simulink model "SPGF_FSK_0000_R2020b"  (R2020b)
settings: Solver=ode4  StartTime=0.0  StopTime=1.4  FixedStep=50e-6/50  RelTol=1e-3  EnableMultiTasking=on
undefined symbols (not defined in the file): D11, Delta
libraries: powerlib x2546, powerlib_meascontrol x183, simulink x24
(part 24 of 34)

== system SPGF_FSK_0000_R2020b/W35/concentrated ==
  Ccs/1 : powerlib/Elements/Series RLC Branch  LConnTagsString=__new0  RConnTagsString=__new0  BranchType=C  Resistance=190  Inductance=1e-3  SetiL0=off  InitialCurrent=0  Capacitance=-C_matrix(1,2)/2  Setx0=off  InitialVoltage=0  Measurements=None
  Ccs/2 : powerlib/Elements/Series RLC Branch  LConnTagsString=__new0  RConnTagsString=__new0  BranchType=C  Resistance=190  Inductance=1e-3  SetiL0=off  InitialCurrent=0  Capacitance=-C_matrix(1,2)/2  Setx0=off  InitialVoltage=0  Measurements=None
  Ccs2/1 : powerlib/Elements/Series RLC Branch  LConnTagsString=__new0  RConnTagsString=__new0  BranchType=C  Resistance=190  Inductance=1e-3  SetiL0=off  InitialCurrent=0  Capacitance=-C_matrix(3,4)/2  Setx0=off  InitialVoltage=0  Measurements=None
  Ccs2/2 : powerlib/Elements/Series RLC Branch  LConnTagsString=__new0  RConnTagsString=__new0  BranchType=C  Resistance=190  Inductance=1e-3  SetiL0=off  InitialCurrent=0  Capacitance=-C_matrix(3,4)/2  Setx0=off  InitialVoltage=0  Measurements=None
  Ccs2/3 : powerlib/Elements/Series RLC Branch  LConnTagsString=__new0  RConnTagsString=__new0  BranchType=R  Resistance=-Rg_matrix(3,4)*2  Inductance=1e-3  SetiL0=off  InitialCurrent=0  Capacitance=Rg_matrix(3,4)*2  Setx0=off  InitialVoltage=0  Measurements=None
  Ccs2/4 : powerlib/Elements/Series RLC Branch  LConnTagsString=__new0  RConnTagsString=__new0  BranchType=R  Resistance=-Rg_matrix(3,4)*2  Inductance=1e-3  SetiL0=off  InitialCurrent=0  Capacitance=Rg_matrix(3,4)*2  Setx0=off  InitialVoltage=0  Measurements=None
  Ccs3/1 : powerlib/Elements/Series RLC Branch  LConnTagsString=__new0  RConnTagsString=__new0  BranchType=C  Resistance=190  Inductance=1e-3  SetiL0=off  InitialCurrent=0  Capacitance=-C_matrix(5,6)/2  Setx0=off  InitialVoltage=0  Measurements=None
  Ccs3/2 : powerlib/Elements/Series RLC Branch  LConnTagsString=__new0  RConnTagsString=__new0  BranchType=C  Resistance=190  Inductance=1e-3  SetiL0=off  InitialCurrent=0  Capacitance=-C_matrix(5,6)/2  Setx0=off  InitialVoltage=0  Measurements=None
  Ccs3/3 : powerlib/Elements/Series RLC Branch  LConnTagsString=__new0  RConnTagsString=__new0  BranchType=R  Resistance=-Rg_matrix(5,6)*2  Inductance=1e-3  SetiL0=off  InitialCurrent=0  Capacitance=-C_matrix(5,6)/2  Setx0=off  InitialVoltage=0  Measurements=None
  Ccs3/4 : powerlib/Elements/Series RLC Branch  LConnTagsString=__new0  RConnTagsString=__new0  BranchType=R  Resistance=-Rg_matrix(5,6)*2  Inductance=1e-3  SetiL0=off  InitialCurrent=0  Capacitance=-C_matrix(5,6)/2  Setx0=off  InitialVoltage=0  Measurements=None
  Csg/2 : powerlib/Elements/Series RLC Branch  LConnTagsString=__new0  RConnTagsString=__new0  BranchType=C  Resistance=190  Inductance=1e-3  SetiL0=off  InitialCurrent=0  Capacitance=( C_matrix(1,2) + C_matrix(2,2) )/2  Setx0=off  InitialVoltage=0  Measurements=None
  Csg1/1 : powerlib/Elements/Series RLC Branch  LConnTagsString=__new0  RConnTagsString=__new0  BranchType=C  Resistance=190  Inductance=1e-3  SetiL0=off  InitialCurrent=0  Capacitance=( C_matrix(1,2) + C_matrix(2,2) )/2  Setx0=off  InitialVoltage=0  Measurements=None
  Csg2/1 : powerlib/Elements/Series RLC Branch  LConnTagsString=__new0  RConnTagsString=__new0  BranchType=C  Resistance=190  Inductance=1e-3  SetiL0=off  InitialCurrent=0  Capacitance=( C_matrix(3,4) + C_matrix(4,4) )/2  Setx0=off  InitialVoltage=0  Measurements=None
  Csg2/2 : powerlib/Elements/Series RLC Branch  LConnTagsString=__new0  RConnTagsString=__new0  BranchType=C  Resistance=190  Inductance=1e-3  SetiL0=off  InitialCurrent=0  Capacitance=( C_matrix(3,4) + C_matrix(4,4) )/2  Setx0=off  InitialVoltage=0  Measurements=None
  Csg3/1 : powerlib/Elements/Series RLC Branch  LConnTagsString=__new0  RConnTagsString=__new0  BranchType=C  Resistance=190  Inductance=1e-3  SetiL0=off  InitialCurrent=0  Capacitance=( C_matrix(5,6) + C_matrix(6,6) ) /2  Setx0=off  InitialVoltage=0  Measurements=None
  Csg3/2 : powerlib/Elements/Series RLC Branch  LConnTagsString=__new0  RConnTagsString=__new0  BranchType=C  Resistance=190  Inductance=1e-3  SetiL0=off  InitialCurrent=0  Capacitance=( C_matrix(5,6) + C_matrix(6,6) ) /2  Setx0=off  InitialVoltage=0  Measurements=None
  Ground{1..4} (4 alike) : powerlib/Elements/Ground  LConnTagsString=a
  RL : powerlib/Elements/Mutual Inductance  LConnTagsString=a|b|c|L4|L5|L6  RConnTagsString=A|B|C|R4|R5|R6  TypeOfMutual=Generalized mutual inductance  NumberOfWindings=6  SelfImpedance1=[1.1 1.1e-03]  SelfImpedance2=[ 1.1 1.1e-03]  ThreeWindings=on  SelfImpedance3=[ 1.1 1.1e-03]  MutualImpedance=[1.0 1.0e-03]  InductanceMatrix=L_matrix  ResistanceMatrix=R_matrix  Measurements=None
      settings: AttributesFormatString=\n
  Rcs*2 : powerlib/Elements/Series RLC Branch  LConnTagsString=__new0  RConnTagsString=__new0  BranchType=R  Resistance=-Rg_matrix(1,2)*2  Inductance=1e-3  SetiL0=off  InitialCurrent=0  Capacitance=Rg_matrix(1,2)*2  Setx0=off  InitialVoltage=0  Measurements=None
  Rgcs1/1 : powerlib/Elements/Series RLC Branch  LConnTagsString=__new0  RConnTagsString=__new0  BranchType=R  Resistance=-Rg_matrix(1,2)*2  Inductance=1e-3  SetiL0=off  InitialCurrent=0  Capacitance=Rg_matrix(1,2)*2  Setx0=off  InitialVoltage=0  Measurements=None
  Rgsg1/1 : powerlib/Elements/Series RLC Branch  LConnTagsString=__new0  RConnTagsString=__new0  BranchType=R  Resistance=(Rg_matrix(4,4)+Rg_matrix(3,4))*2  Inductance=1e-3  SetiL0=off  InitialCurrent=0  Capacitance=Rg_matrix(1,2)*2  Setx0=off  InitialVoltage=0  Measurements=None
  Rgsg1/2 : powerlib/Elements/Series RLC Branch  LConnTagsString=__new0  RConnTagsString=__new0  BranchType=R  Resistance=(Rg_matrix(2,2)+Rg_matrix(1,2))*2  Inductance=1e-3  SetiL0=off  InitialCurrent=0  Capacitance=Rg_matrix(1,2)*2  Setx0=off  InitialVoltage=0  Measurements=None
  Rgsg1/3 : powerlib/Elements/Series RLC Branch  LConnTagsString=__new0  RConnTagsString=__new0  BranchType=R  Resistance=(Rg_matrix(4,4)+Rg_matrix(3,4))*2  Inductance=1e-3  SetiL0=off  InitialCurrent=0  Capacitance=Rg_matrix(1,2)*2  Setx0=off  InitialVoltage=0  Measurements=None
  Rgsg1/4 : powerlib/Elements/Series RLC Branch  LConnTagsString=__new0  RConnTagsString=__new0  BranchType=R  Resistance=(Rg_matrix(2,2)+Rg_matrix(1,2))*2  Inductance=1e-3  SetiL0=off  InitialCurrent=0  Capacitance=Rg_matrix(1,2)*2  Setx0=off  InitialVoltage=0  Measurements=None
  Rsg*2 : powerlib/Elements/Series RLC Branch  LConnTagsString=__new0  RConnTagsString=__new0  BranchType=R  Resistance=(Rg_matrix(6,6)+Rg_matrix(5,6))*2  Inductance=1e-3  SetiL0=off  InitialCurrent=0  Capacitance=Rg_matrix(1,2)*2  Setx0=off  InitialVoltage=0  Measurements=None
  Rsg1/1 : powerlib/Elements/Series RLC Branch  LConnTagsString=__new0  RConnTagsString=__new0  BranchType=R  Resistance=(Rg_matrix(6,6)+Rg_matrix(5,6))*2  Inductance=1e-3  SetiL0=off  InitialCurrent=0  Capacitance=Rg_matrix(1,2)*2  Setx0=off  InitialVoltage=0  Measurements=None
  A : PMIOPort  Side=Left
  B : PMIOPort  Port=2  Side=Left
  C : PMIOPort  Port=3  Side=Left
  a : PMIOPort  Port=4  Side=Right
  b : PMIOPort  Port=5  Side=Right
  c : PMIOPort  Port=6  Side=Right
  connections:
  RL/LConn6 -- Ground3/LConn1 -- Rgsg1/2/LConn1 -- Csg/2/LConn1 -- Rcs*2/LConn1 -- Ccs/2/LConn1 -- RL/LConn2 -- RL/LConn4 -- Rgsg1/1/LConn1 -- Csg2/2/LConn1 -- Ccs2/3/LConn1 -- Ccs2/2/LConn1 -- Rsg*2/LConn1 -- Csg3/2/LConn1 -- Ccs3/3/LConn1 -- Ccs3/2/LConn1
  Rsg1/1/RConn1 -- Rgsg1/3/RConn1 -- Rgsg1/4/RConn1 -- Csg3/1/RConn1 -- Csg2/1/RConn1 -- Ground2/LConn1 -- Csg1/1/RConn1
  Rgsg1/3/LConn1 -- Ccs2/4/LConn1 -- Csg2/1/LConn1 -- Ccs2/1/LConn1 -- RL/RConn4 -- Rgsg1/4/LConn1 -- Rgcs1/1/LConn1 -- Csg1/1/LConn1 -- Ccs/1/LConn1 -- RL/RConn2 -- Ground4/LConn1 -- RL/RConn6 -- Ccs3/1/LConn1 -- Rsg1/1/LConn1 -- Ccs3/4/LConn1 -- Csg3/1/LConn1
  Rsg*2/RConn1 -- Rgsg1/1/RConn1 -- Rgsg1/2/RConn1 -- Csg3/2/RConn1 -- Csg2/2/RConn1 -- Ground1/LConn1 -- Csg/2/RConn1
  a/RConn1 -- RL/RConn1 -- Rgcs1/1/RConn1 -- Ccs/1/RConn1
  b/RConn1 -- RL/RConn3 -- Ccs2/4/RConn1 -- Ccs2/1/RConn1
  Ccs3/1/RConn1 -- c/RConn1 -- RL/RConn5 -- Ccs3/4/RConn1
  RL/LConn1 -- A/RConn1 -- Rcs*2/RConn1 -- Ccs/2/RConn1
  RL/LConn3 -- B/RConn1 -- Ccs2/3/RConn1 -- Ccs2/2/RConn1
  Ccs3/2/RConn1 -- C/RConn1 -- RL/LConn5 -- Ccs3/3/RConn1

== system SPGF_FSK_0000_R2020b/W41/DPL ==
  Ccs2/1 : powerlib/Elements/Series RLC Branch  LConnTagsString=__new0  RConnTagsString=__new0  BranchType=R  Resistance=-Rg_matrix(3,4)*2  Inductance=1e-3  SetiL0=off  InitialCurrent=0  Capacitance=Rg_matrix(3,4)*2  Setx0=off  InitialVoltage=0  Measurements=None
  Ccs2/3 : powerlib/Elements/Series RLC Branch  LConnTagsString=__new0  RConnTagsString=__new0  BranchType=R  Resistance=-Rg_matrix(3,4)*2  Inductance=1e-3  SetiL0=off  InitialCurrent=0  Capacitance=Rg_matrix(3,4)*2  Setx0=off  InitialVoltage=0  Measurements=None
  Ccs3/1 : powerlib/Elements/Series RLC Branch  LConnTagsString=__new0  RConnTagsString=__new0  BranchType=R  Resistance=-Rg_matrix(5,6)*2  Inductance=1e-3  SetiL0=off  InitialCurrent=0  Capacitance=-C_matrix(5,6)/2  Setx0=off  InitialVoltage=0  Measurements=None
  Ccs3/3 : powerlib/Elements/Series RLC Branch  LConnTagsString=__new0  RConnTagsString=__new0  BranchType=R  Resistance=-Rg_matrix(5,6)*2  Inductance=1e-3  SetiL0=off  InitialCurrent=0  Capacitance=-C_matrix(5,6)/2  Setx0=off  InitialVoltage=0  Measurements=None
  DPL : powerlib/Elements/Distributed Parameters Line  Phases=6  Length=LineLength  Frequency=Frequency  Resistance=R_matrix  Inductance=L_matrix  Capacitance=C_matrix  x1=[-2.1e-05 -1.17011401823538 0 0 0 0 0;-2.05e-05 -1.17045633373084 0 0 0 0 0;-2e-05 -1.17079862034645 0 0 0 0 0;-1.95e-05 -1.17114087807377 0 0 0 0 0;-1.9e-05 -1.17148310690434 0 0 0 0 0;-1.85e-05 -1.17182530682973 0 0 0 0 0;-1.8e-05 -1.17216747784148 0 0 0 0 0;-1.75e-05 -1.17250961993116 0 0 0 0 0;-1.7e-05 -1.17285173309033 0 0 0 0 0;-1.65e-05 -1.17319381731054 0 0 0 0 0;-1.6e-05 -1.17353587258335 0 0 0 0 0;-1.55e-05 -1.17387789890033 0 0 0 0 0;-1.5e-05 -1.17421989625302 0 0 0 0 0;-1.45e-05 -1.17456186463301 0 0 0 0 0;-1.4e-05 -1.17490380403184 0 0 0 0 0;-1.35e-05 -1.17524571444108 0 0 0 0 0;-1.3e-05 -1.1755875958523 0 0 0 0 0;-1.25e-05 -1.17592944825706 0 0 0 0 0;-1.2e-05 -1.17627127164692 0 0 0 0 0;-1.15e-05 -1.17661306601345 0 0 0 0 0;-1.1e-05 -1.17695483134822 0 0 0 0 0;-1.05e-05 -1.17729656764278 0 0 0 0 0;-1e-05 -1.17763827488873 0 0 0 0 0;-9.5e-06 -1.17797995307761 0 0 0 0 0;-9e-06 -1.178321602201 0 0 0 0 0;-8.5e-06 -1.17866322225047 0 0 0 0 0;-8e-06 -1.17900481321759 0 0 0 0 0;-7.5e-06 -1.17934637509394 0 0 0 0 0;-7e-06 -1.17968790787108 0 0 0 0 0;-6.5e-06 -1.18002941154058 0 0 0 0 0;-6e-06 -1.18037088609403 0 0 0 0 0;-5.5e-06 -1.180712331523 0 0 0 0 0;-5e-06 -1.18105374781905 0 0 0 0 0;-4.5e-06 -1.18139513497377 0 -12.6730292405326 0 0 0;-4e-06 -1.18173649297874 5125.65658858161 -12.6767469395124 -2807.98045194031 0 0;-3.5e-06 -1.18207782182552 5127.08623497509 -12.6804643257059 -2808.76365289363 4986.53730385231 -9096.55192111757;-3e-06 -1.18241912150571 5128.51575486278 -12.6841813990215 -2809.5467845435 4986.09584905122 -9095.7466094806;-2.5e-06 -1.18276039201087 5129.94514820942 -12.6878981593675 -2810.32984687057 4985.65427122314 -9094.94107341507;-2e-06 -1.18310163333259 5131.37441497974 -12.6916146066521 -2811.11283985553 4985.21257037897 -9094.13531294087;-1.5e-06 -1.18344284546245 5132.80355513847 -12.6953307407837 -2811.89576347907 4984.77074652961 -9093.32932807787;-1e-06 -1.18378402839202 5134.23256865034 -12.6990465616706 -2812.67861772185 4984.32879968597 -9092.52311884597;-5e-07 -1.1841251821129 5135.66145548011 -12.7027620692211 -2813.46140256458 4983.88672985894 -9091.71668526505]  x2=[-2.1e-05 -1.16992811610187 0 0 0 0 0;-2.05e-05 -1.17027211355506 0 0 0 0 0;-2e-05 -1.17061608213293 0 0 0 0 0;-1.95e-05 -1.17096002182702 0 0 0 0 0;-1.9e-05 -1.17130393262882 0 0 0 0 0;-1.85e-05 -1.17164781452986 0 0 0 0 0;-1.8e-05 -1.17199166752164 0 0 0 0 0;-1.75e-05 -1.17233549159569 0 0 0 0 0;-1.7e-05 -1.17267928674353 0 0 0 0 0;-1.65e-05 -1.17302305295666 0 0 0 0 0;-1.6e-05 -1.1733667902266 0 0 0 0 0;-1.55e-05 -1.17371049854489 0 0 0 0 0;-1.5e-05 -1.17405417790302 0 0 0 0 0;-1.45e-05 -1.17439782829253 0 0 0 0 0;-1.4e-05 -1.17474144970494 0 0 0 0 0;-1.35e-05 -1.17508504213176 0 0 0 0 0;-1.3e-05 -1.17542860556452 0 0 0 0 0;-1.25e-05 -1.17577213999474 0 0 0 0 0;-1.2e-05 -1.17611564541395 0 0 0 0 0;-1.15e-05 -1.17645912181367 0 0 0 0 0;-1.1e-05 -1.17680256918542 0 0 0 0 0;-1.05e-05 -1.17714598752073 0 0 0 0 0;-1e-05 -1.17748937681113 0 0 0 0 0;-9.5e-06 -1.17783273704815 0 0 0 0 0;-9e-06 -1.1781760682233 0 0 0 0 0;-8.5e-06 -1.17851937032813 0 0 0 0 0;-8e-06 -1.17886264335416 0 0 0 0 0;-7.5e-06 -1.17920588729292 0 0 0 0 0;-7e-06 -1.17954910213593 0 0 0 0 0;-6.5e-06 -1.17989228787475 0 0 0 0 0;-6e-06 -1.18023544450088 0 0 0 0 0;-5.5e-06 -1.18057857200588 0 0 0 0 0;-5e-06 -1.18092167038126 0 0 0 0 0;-4.5e-06 -1.18126473961857 0 -12.6639649895814 0 0 0;-4e-06 -1.18160777970934 5132.06710220299 -12.6677056982318 -2811.49231360161 0 0;-3.5e-06 -1.18195079064511 5133.49952711031 -12.6714460943191 -2812.27703670385 4995.83428251018 -9113.51167573637;-3e-06 -1.18229377241741 5134.9318253536 -12.675186177751 -2813.06169041594 4995.39247476773 -9112.70572025595;-2.5e-06 -1.18263672501778 5136.36399689754 -12.6789259484352 -2813.84627471851 4994.95054376891 -9111.89953992853;-2e-06 -1.18297964843776 5137.79604170677 -12.6826654062795 -2814.6307895922 4994.50848952462 -9111.09313477399;-1.5e-06 -1.18332254266889 5139.22795974596 -12.6864045511915 -2815.41523501767 4994.06631204578 -9110.28650481225;-1e-06 -1.18366540770271 5140.65975097979 -12.6901433830791 -2816.19961097555 4993.62401134329 -9109.4796500632;-5e-07 -1.18400824353075 5142.09141537292 -12.6938819018499 -2816.98391744649 4993.18158742807 -9108.67257054674]  x3=[-2.1e-05 0.0021659765455351 0 0 0 0 0;-2.05e-05 0.00216349910489419 0 0 0 0 0;-2e-05 0.00216102161087109 0 0 0 0 0;-1.95e-05 0.00215854406352692 0 0 0 0 0;-1.9e-05 0.0021560664629228 0 0 0 0 0;-1.85e-05 0.00215358880911988 0 0 0 0 0;-1.8e-05 0.00215111110217928 0 0 0 0 0;-1.75e-05 0.00214863334216215 0 0 0 0 0;-1.7e-05 0.00214615552912961 0 0 0 0 0;-1.65e-05 0.00214367766314281 0 0 0 0 0;-1.6e-05 0.00214119974426288 0 0 0 0 0;-1.55e-05 0.00213872177255097 0 0 0 0 0;-1.5e-05 0.00213624374806821 0 0 0 0 0;-1.45e-05 0.00213376567087575 0 0 0 0 0;-1.4e-05 0.00213128754103473 0 0 0 0 0;-1.35e-05 0.0021288093586063 0 0 0 0 0;-1.3e-05 0.0021263311236516 0 0 0 0 0;-1.25e-05 0.00212385283623179 0 0 0 0 0;-1.2e-05 0.00212137449640801 0 0 0 0 0;-1.15e-05 0.00211889610424141 0 0 0 0 0;-1.1e-05 0.00211641765979314 0 0 0 0 0;-1.05e-05 0.00211393916312437 0 0 0 0 0;-1e-05 0.00211146061429623 0 0 0 0 0;-9.5e-06 0.00210898201336989 0 0 0 0 0;-9e-06 0.00210650336040651 0 0 0 0 0;-8.5e-06 0.00210402465546724 0 0 0 0 0;-8e-06 0.00210154589861324 0 0 0 0 0;-7.5e-06 0.00209906708990568 0 0 0 0 0;-7e-06 0.00209658822940571 0 0 0 0 0;-6.5e-06 0.0020941093171745 0 0 0 0 0;-6e-06 0.00209163035327322 0 0 0 0 0;-5.5e-06 0.00208915133776302 0 0 0 0 0;-5e-06 0.00208667227070509 0 0 0 0 0;-4.5e-06 0.00208419315216057 0 -0.812876199765621 0 0 0;-4e-06 0.00208171398219065 38.0377374888532 -0.813270853696157 -268.727129623902 0 0;-3.5e-06 0.0020792347608565 38.0761261833707 -0.81366548756004 -268.805479923023 527.730053815073 -266.618450812591;-3e-06 0.00207675548821929 38.1145139383975 -0.814060101347531 -268.883823589634 527.685899314859 -266.61014142652;-2.5e-06 0.00207427616434019 38.1529007529863 -0.814454695048894 -268.962160621803 527.641731794517 -266.601825462107;-2e-06 0.00207179678928038 38.1912866261901 -0.814849268654394 -269.040491017597 527.597551255138 -266.593502919558;-1.5e-06 0.00206931736310103 38.2296715570616 -0.815243822154293 -269.118814775083 527.55335769781 -266.585173799078;-1e-06 0.00206683788586332 38.2680555446538 -0.815638355538858 -269.197131892328 527.509151123626 -266.576838100872;-5e-07 0.00206435835762843 38.3064385880195 -0.816032868798352 -269.2754423674 527.464931533674 -266.568495825147]  x4=[-2.1e-05 -0.0162868088719323 0 0 0 0 0;-2.05e-05 -0.0162885056488091 0 0 0 0 0;-2e-05 -0.0162902020237832 0 0 0 0 0;-1.95e-05 -0.0162918979968126 0 0 0 0 0;-1.9e-05 -0.0162935935678555 0 0 0 0 0;-1.85e-05 -0.0162952887368702 0 0 0 0 0;-1.8e-05 -0.0162969835038147 0 0 0 0 0;-1.75e-05 -0.0162986778686473 0 0 0 0 0;-1.7e-05 -0.0163003718313261 0 0 0 0 0;-1.65e-05 -0.0163020653918093 0 0 0 0 0;-1.6e-05 -0.0163037585500553 0 0 0 0 0;-1.55e-05 -0.0163054513060221 0 0 0 0 0;-1.5e-05 -0.016307143659668 0 0 0 0 0;-1.45e-05 -0.0163088356109512 0 0 0 0 0;-1.4e-05 -0.0163105271598301 0 0 0 0 0;-1.35e-05 -0.0163122183062629 0 0 0 0 0;-1.3e-05 -0.0163139090502078 0 0 0 0 0;-1.25e-05 -0.0163155993916231 0 0 0 0 0;-1.2e-05 -0.0163172893304672 0 0 0 0 0;-1.15e-05 -0.0163189788666983 0 0 0 0 0;-1.1e-05 -0.0163206680002747 0 0 0 0 0;-1.05e-05 -0.0163223567311548 0 0 0 0 0;-1e-05 -0.0163240450592968 0 0 0 0 0;-9.5e-06 -0.0163257329846593 0 0 0 0 0;-9e-06 -0.0163274205072003 0 0 0 0 0;-8.5e-06 -0.0163291076268785 0 0 0 0 0;-8e-06 -0.016330794343652 0 0 0 0 0;-7.5e-06 -0.0163324806574794 0 0 0 0 0;-7e-06 -0.0163341665683189 0 0 0 0 0;-6.5e-06 -0.0163358520761291 0 0 0 0 0;-6e-06 -0.0163375371808682 0 0 0 0 0;-5.5e-06 -0.0163392218824948 0 0 0 0 0;-5e-06 -0.0163409061809673 0 0 0 0 0;-4.5e-06 -0.016342590076244 0 -1.04999882623992 0 0 0;-4e-06 -0.0163442735682835 98.9043685697564 -1.05015338706581 -242.003028604929 0 0;-3.5e-06 -0.0163459566570442 98.9042385142842 -1.05030792198022 -242.067368447992 442.924329707491 -18.8617468671821;-3e-06 -0.0163476393424846 98.9041060184477 -1.05046243097931 -242.131702318283 442.882704413754 -18.8448242630082;-2.5e-06 -0.0163493216245632 98.9039710822503 -1.05061691405928 -242.196030214214 442.841068192324 -18.8279011938569;-2e-06 -0.0163510035032384 98.9038337056951 -1.05077137121631 -242.260352134197 442.79942104423 -18.8109776601457;-1.5e-06 -0.0163526849784688 98.9036938887857 -1.05092580244661 -242.324668076645 442.757762970497 -18.7940536622922;-1e-06 -0.0163543660502129 98.9035516315254 -1.05108020774635 -242.388978039972 442.716093972154 -18.7771292007141;-5e-07 -0.0163560467184291 98.9034069339179 -1.05123458711172 -242.453282022591 442.67441405023 -18.7602042758289]  x5=2.07854383214439e-05  V1=ones(3,3)  V2=ones(3,3)  I1=ones(3,3)  I2=ones(3,3)  nHarmo=1  Measurements=None  Decoupling=off  VsMag0=0  VrMag0=0  VsAngle0=0  VrAngle0=0  IsMag0=0  IrMag0=0  IsAngle0=0  IrAngle0=0
  Ground{1..4} (4 alike) : powerlib/Elements/Ground  LConnTagsString=a
  Rcs*1 : powerlib/Elements/Series RLC Branch  LConnTagsString=__new0  RConnTagsString=__new0  BranchType=R  Resistance=-Rg_matrix(1,2)*2  Inductance=1e-3  SetiL0=off  InitialCurrent=0  Capacitance=Rg_matrix(1,2)*2  Setx0=off  InitialVoltage=0  Measurements=None
  Rcs*2 : powerlib/Elements/Series RLC Branch  LConnTagsString=__new0  RConnTagsString=__new0  BranchType=R  Resistance=-Rg_matrix(1,2)*2  Inductance=1e-3  SetiL0=off  InitialCurrent=0  Capacitance=Rg_matrix(1,2)*2  Setx0=off  InitialVoltage=0  Measurements=None
  Rgsg1/1 : powerlib/Elements/Series RLC Branch  LConnTagsString=__new0  RConnTagsString=__new0  BranchType=R  Resistance=(Rg_matrix(4,4)+Rg_matrix(3,4))*2  Inductance=1e-3  SetiL0=off  InitialCurrent=0  Capacitance=Rg_matrix(1,2)*2  Setx0=off  InitialVoltage=0  Measurements=None
  Rgsg1/2 : powerlib/Elements/Series RLC Branch  LConnTagsString=__new0  RConnTagsString=__new0  BranchType=R  Resistance=(Rg_matrix(2,2)+Rg_matrix(1,2))*2  Inductance=1e-3  SetiL0=off  InitialCurrent=0  Capacitance=Rg_matrix(1,2)*2  Setx0=off  InitialVoltage=0  Measurements=None
  Rgsg1/3 : powerlib/Elements/Series RLC Branch  LConnTagsString=__new0  RConnTagsString=__new0  BranchType=R  Resistance=(Rg_matrix(4,4)+Rg_matrix(3,4))*2  Inductance=1e-3  SetiL0=off  InitialCurrent=0  Capacitance=Rg_matrix(1,2)*2  Setx0=off  InitialVoltage=0  Measurements=None
  Rgsg1/4 : powerlib/Elements/Series RLC Branch  LConnTagsString=__new0  RConnTagsString=__new0  BranchType=R  Resistance=(Rg_matrix(2,2)+Rg_matrix(1,2))*2  Inductance=1e-3  SetiL0=off  InitialCurrent=0  Capacitance=Rg_matrix(1,2)*2  Setx0=off  InitialVoltage=0  Measurements=None
  Rsg*1 : powerlib/Elements/Series RLC Branch  LConnTagsString=__new0  RConnTagsString=__new0  BranchType=R  Resistance=(Rg_matrix(6,6)+Rg_matrix(5,6))*2  Inductance=1e-3  SetiL0=off  InitialCurrent=0  Capacitance=Rg_matrix(1,2)*2  Setx0=off  InitialVoltage=0  Measurements=None
  Rsg*2 : powerlib/Elements/Series RLC Branch  LConnTagsString=__new0  RConnTagsString=__new0  BranchType=R  Resistance=(Rg_matrix(6,6)+Rg_matrix(5,6))*2  Inductance=1e-3  SetiL0=off  InitialCurrent=0  Capacitance=Rg_matrix(1,2)*2  Setx0=off  InitialVoltage=0  Measurements=None
  A : PMIOPort  Side=Left
  B : PMIOPort  Port=2  Side=Left
  C : PMIOPort  Port=3  Side=Left
  a : PMIOPort  Port=4  Side=Right
  b : PMIOPort  Port=5  Side=Right
  c : PMIOPort  Port=6  Side=Right
  connections:
  A/RConn1 -- DPL/LConn1 -- Rcs*2/RConn1
  B/RConn1 -- DPL/LConn3 -- Ccs2/3/RConn1
  C/RConn1 -- DPL/LConn5 -- Ccs3/3/RConn1
  Rgsg1/2/RConn1 -- Rsg*2/RConn1 -- Rgsg1/1/RConn1 -- Ground2/LConn1
  DPL/LConn2 -- Rcs*2/LConn1 -- Rgsg1/2/LConn1 -- DPL/LConn4 -- Ccs2/3/LConn1 -- Rgsg1/1/LConn1 -- DPL/LConn6 -- Rsg*2/LConn1 -- Ccs3/3/LConn1 -- Ground3/LConn1
  Rgsg1/3/RConn1 -- Rsg*1/RConn1 -- Rgsg1/4/RConn1 -- Ground1/LConn1
  Rgsg1/3/LConn1 -- Ccs2/1/LConn1 -- DPL/RConn4 -- DPL/RConn2 -- Rgsg1/4/LConn1 -- Rcs*1/LConn1 -- Rsg*1/LConn1 -- Ccs3/1/LConn1 -- DPL/RConn6 -- Ground4/LConn1
  Rcs*1/RConn1 -- DPL/RConn1 -- a/RConn1
  DPL/RConn3 -- Ccs2/1/RConn1 -- b/RConn1
  DPL/RConn5 -- Ccs3/1/RConn1 -- c/RConn1

== system SPGF_FSK_0000_R2020b/W41/Pi ==
  Ground{,1..8} (9 alike) : powerlib/Elements/Ground  LConnTagsString=a
  Series RLC Branch{,1..2,27..28,33} (6 alike) : powerlib/Elements/Series RLC Branch  LConnTagsString=__new0  RConnTagsString=__new0  BranchType=RL  Resistance=R/2  Inductance=L/2  SetiL0=off  InitialCurrent=0  Capacitance=1e-6  Setx0=off  InitialVoltage=0  Measurements=None
  Series RLC Branch{10..11,13,29..30,32} (6 alike) : powerlib/Elements/Series RLC Branch  LConnTagsString=__new0  RConnTagsString=__new0  BranchType=R  Resistance=Rfg*4  Inductance=L/2  SetiL0=off  InitialCurrent=0  Capacitance=1e-6  Setx0=off  InitialVoltage=0  Measurements=None
  Series RLC Branch{9,12,14,31,40..41} (6 alike) : powerlib/Elements/Series RLC Branch  LConnTagsString=__new0  RConnTagsString=__new0  BranchType=C  Resistance=R/2  Inductance=L/2  SetiL0=off  InitialCurrent=0  Capacitance=Cfg*0.25  Setx0=off  InitialVoltage=0  Measurements=None
  Series RLC Branch15 : powerlib/Elements/Series RLC Branch  LConnTagsString=__new0  RConnTagsString=__new0  BranchType=R  Resistance=Rfg*2  Inductance=L/2  SetiL0=off  InitialCurrent=0  Capacitance=1e-6  Setx0=off  InitialVoltage=0  Measurements=None
  Series RLC Branch16 : powerlib/Elements/Series RLC Branch  LConnTagsString=__new0  RConnTagsString=__new0  BranchType=R  Resistance=Rfg*2  Inductance=L/2  SetiL0=off  InitialCurrent=0  Capacitance=1e-6  Setx0=off  InitialVoltage=0  Measurements=None
  Series RLC Branch17 : powerlib/Elements/Series RLC Branch  LConnTagsString=__new0  RConnTagsString=__new0  BranchType=C  Resistance=R/2  Inductance=L/2  SetiL0=off  InitialCurrent=0  Capacitance=Cfg*0.5  Setx0=off  InitialVoltage=0  Measurements=None
  Series RLC Branch18 : powerlib/Elements/Series RLC Branch  LConnTagsString=__new0  RConnTagsString=__new0  BranchType=R  Resistance=Rfg*2  Inductance=L/2  SetiL0=off  InitialCurrent=0  Capacitance=1e-6  Setx0=off  InitialVoltage=0  Measurements=None
  Series RLC Branch19 : powerlib/Elements/Series RLC Branch  LConnTagsString=__new0  RConnTagsString=__new0  BranchType=C  Resistance=R/2  Inductance=L/2  SetiL0=off  InitialCurrent=0  Capacitance=Cfg*0.5  Setx0=off  InitialVoltage=0  Measurements=None
  Series RLC Branch20 : powerlib/Elements/Series RLC Branch  LConnTagsString=__new0  RConnTagsString=__new0  BranchType=C  Resistance=R/2  Inductance=L/2  SetiL0=off  InitialCurrent=0  Capacitance=Cmf*0.5  Setx0=off  InitialVoltage=0  Measurements=None
  Series RLC Branch21 : powerlib/Elements/Series RLC Branch  LConnTagsString=__new0  RConnTagsString=__new0  BranchType=R  Resistance=Rmf*2  Inductance=L/2  SetiL0=off  InitialCurrent=0  Capacitance=1e-6  Setx0=off  InitialVoltage=0  Measurements=None
  Series RLC Branch22 : powerlib/Elements/Series RLC Branch  LConnTagsString=__new0  RConnTagsString=__new0  BranchType=C  Resistance=R/2  Inductance=L/2  SetiL0=off  InitialCurrent=0  Capacitance=Cmf*0.5  Setx0=off  InitialVoltage=0  Measurements=None
  Series RLC Branch23 : powerlib/Elements/Series RLC Branch  LConnTagsString=__new0  RConnTagsString=__new0  BranchType=R  Resistance=Rmf*2  Inductance=L/2  SetiL0=off  InitialCurrent=0  Capacitance=1e-6  Setx0=off  InitialVoltage=0  Measurements=None
  Series RLC Branch24 : powerlib/Elements/Series RLC Branch  LConnTagsString=__new0  RConnTagsString=__new0  BranchType=C  Resistance=R/2  Inductance=L/2  SetiL0=off  InitialCurrent=0  Capacitance=Cmf*0.5  Setx0=off  InitialVoltage=0  Measurements=None
  Series RLC Branch25 : powerlib/Elements/Series RLC Branch  LConnTagsString=__new0  RConnTagsString=__new0  BranchType=R  Resistance=Rmf*2  Inductance=L/2  SetiL0=off  InitialCurrent=0  Capacitance=1e-6  Setx0=off  InitialVoltage=0  Measurements=None
  Series RLC Branch26 : powerlib/Elements/Series RLC Branch  LConnTagsString=__new0  RConnTagsString=__new0  BranchType=C  Resistance=R/2  Inductance=L/2  SetiL0=off  InitialCurrent=0  Capacitance=Cfg*0.5  Setx0=off  InitialVoltage=0  Measurements=None
  Series RLC Branch{3,5,7,34,36,38} (6 alike) : powerlib/Elements/Series RLC Branch  LConnTagsString=__new0  RConnTagsString=__new0  BranchType=C  Resistance=R/2  Inductance=L/2  SetiL0=off  InitialCurrent=0  Capacitance=Cmf*0.25  Setx0=off  InitialVoltage=0  Measurements=None
  Series RLC Branch{4,6,8,35,37,39} (6 alike) : powerlib/Elements/Series RLC Branch  LConnTagsString=__new0  RConnTagsString=__new0  BranchType=R  Resistance=Rmf*4  Inductance=L/2  SetiL0=off  InitialCurrent=0  Capacitance=1e-6  Setx0=off  InitialVoltage=0  Measurements=None
  A : PMIOPort  Side=Left
  B : PMIOPort  Port=2  Side=Left
  C : PMIOPort  Port=3  Side=Left
  a : PMIOPort  Port=4  Side=Right
  b : PMIOPort  Port=5  Side=Right
  c : PMIOPort  Port=6  Side=Right
  connections:
  Series RLC Branch12/LConn1 -- Series RLC Branch11/LConn1 -- Series RLC Branch5/LConn1 -- Series RLC Branch6/LConn1 -- B/RConn1 -- Series RLC Branch4/RConn1 -- Series RLC Branch3/RConn1 -- Series RLC Branch1/LConn1
  Series RLC Branch13/LConn1 -- A/RConn1 -- Series RLC Branch4/LConn1 -- Series RLC Branch3/LConn1 -- Series RLC Branch7/LConn1 -- Series RLC Branch8/LConn1 -- Series RLC Branch/LConn1 -- Series RLC Branch14/LConn1
  Series RLC Branch9/LConn1 -- Series RLC Branch2/LConn1 -- Series RLC Branch8/RConn1 -- Series RLC Branch7/RConn1 -- C/RConn1 -- Series RLC Branch5/RConn1 -- Series RLC Branch6/RConn1 -- Series RLC Branch10/LConn1
  Series RLC Branch9/RConn1 -- Ground/LConn1 -- Series RLC Branch10/RConn1
  Series RLC Branch12/RConn1 -- Series RLC Branch11/RConn1 -- Ground1/LConn1
  Series RLC Branch13/RConn1 -- Series RLC Branch14/RConn1 -- Ground2/LConn1
  Series RLC Branch17/LConn1 -- Series RLC Branch16/LConn1 -- Series RLC Branch28/LConn1 -- Series RLC Branch1/RConn1 -- Series RLC Branch23/LConn1 -- Series RLC Branch22/LConn1 -- Series RLC Branch20/RConn1 -- Series RLC Branch21/RConn1
  Series RLC Branch21/LConn1 -- Series RLC Branch20/LConn1 -- Series RLC Branch/RConn1 -- Series RLC Branch27/LConn1 -- Series RLC Branch19/LConn1 -- Series RLC Branch18/LConn1 -- Series RLC Branch24/LConn1 -- Series RLC Branch25/LConn1
  Series RLC Branch26/LConn1 -- Series RLC Branch15/LConn1 -- Series RLC Branch2/RConn1 -- Series RLC Branch33/LConn1 -- Series RLC Branch25/RConn1 -- Series RLC Branch24/RConn1 -- Series RLC Branch22/RConn1 -- Series RLC Branch23/RConn1
  Series RLC Branch26/RConn1 -- Series RLC Branch15/RConn1 -- Ground3/LConn1
  Ground4/LConn1 -- Series RLC Branch17/RConn1 -- Series RLC Branch16/RConn1
  Ground5/LConn1 -- Series RLC Branch18/RConn1 -- Series RLC Branch19/RConn1
  Series RLC Branch31/LConn1 -- b/RConn1 -- Series RLC Branch35/RConn1 -- Series RLC Branch34/RConn1 -- Series RLC Branch36/LConn1 -- Series RLC Branch37/LConn1 -- Series RLC Branch28/RConn1 -- Series RLC Branch30/LConn1
  Series RLC Branch34/LConn1 -- a/RConn1 -- Series RLC Branch41/LConn1 -- Series RLC Branch32/LConn1 -- Series RLC Branch38/LConn1 -- Series RLC Branch39/LConn1 -- Series RLC Branch27/RConn1 -- Series RLC Branch35/LConn1
  Series RLC Branch29/LConn1 -- Series RLC Branch36/RConn1 -- Series RLC Branch37/RConn1 -- c/RConn1 -- Series RLC Branch39/RConn1 -- Series RLC Branch38/RConn1 -- Series RLC Branch33/RConn1 -- Series RLC Branch40/LConn1
  Series RLC Branch29/RConn1 -- Series RLC Branch40/RConn1 -- Ground6/LConn1
  Series RLC Branch31/RConn1 -- Series RLC Branch30/RConn1 -- Ground7/LConn1
  Series RLC Branch32/RConn1 -- Series RLC Branch41/RConn1 -- Ground8/LConn1

== system SPGF_FSK_0000_R2020b/W41/Q ==
  breaker : Subsystem  Commented=on  mask{SwitchA=on, SwitchB=on, SwitchC=on, InitialStatus=[0 0 0], BreakerResistance=0.0001, SnubberResistance=1e6, SnubberCapacitance=inf, TransitionTimes=[0.2], ShiftTimes=[0 0.02 0.025]}
      mask prompts: SwitchA "Switching of phase A"; SwitchB "Switching of phase B"; SwitchC "Switching of phase C"; InitialStatus "Initial status of phase breaker [A, B, C]"; BreakerResistance "Breaker resistance Ron (ohms) :"; SnubberResistance "Snubbers resistance Rp (ohms) :"; SnubberCapacitance "Snubbers capacitance Cp (F) :"; TransitionTimes "Transition times (s) :"; ShiftTimes "Time differences for switch [tA, tB, tC] (s) :"
      mask init: same as SPGF_FSK_0000_R2020b/Feed/Q/breaker
      mask Display:
      | % port_label('input',1,'Iabc');
      | 
      | port_label('lconn',1,'A');
      | port_label('lconn',2,'B');
      | port_label('lconn',3,'C');
      | 
      | port_label('rconn',1,'a');
      | port_label('rconn',2,'b');
      | port_label('rconn',3,'c');
      | 
      | disp('   Q    ');
  meas : Subsystem
  shunt : Subsystem
  A : PMIOPort  Side=Right
  B : PMIOPort  Port=2  Side=Right
  C : PMIOPort  Port=3  Side=Right
  a : PMIOPort  Port=4  Side=Left
  b : PMIOPort  Port=5  Side=Left
  c : PMIOPort  Port=6  Side=Left
  connections:
  shunt/LConn3 -- breaker/LConn3 -- C/RConn1
  shunt/LConn2 -- breaker/LConn2 -- B/RConn1
  A/RConn1 -- breaker/LConn1 -- shunt/LConn1
  meas/RConn1 -- a/RConn1
  meas/RConn2 -- b/RConn1
  meas/RConn3 -- c/RConn1
  meas/LConn3 -- breaker/RConn3 -- shunt/RConn3
  meas/LConn2 -- breaker/RConn2 -- shunt/RConn2
  meas/LConn1 -- breaker/RConn1 -- shunt/RConn1

== system SPGF_FSK_0000_R2020b/W41/concentrated ==
  Ccs/1 : powerlib/Elements/Series RLC Branch  LConnTagsString=__new0  RConnTagsString=__new0  BranchType=C  Resistance=190  Inductance=1e-3  SetiL0=off  InitialCurrent=0  Capacitance=-C_matrix(1,2)/2  Setx0=off  InitialVoltage=0  Measurements=None
  Ccs/2 : powerlib/Elements/Series RLC Branch  LConnTagsString=__new0  RConnTagsString=__new0  BranchType=C  Resistance=190  Inductance=1e-3  SetiL0=off  InitialCurrent=0  Capacitance=-C_matrix(1,2)/2  Setx0=off  InitialVoltage=0  Measurements=None
  Ccs2/1 : powerlib/Elements/Series RLC Branch  LConnTagsString=__new0  RConnTagsString=__new0  BranchType=C  Resistance=190  Inductance=1e-3  SetiL0=off  InitialCurrent=0  Capacitance=-C_matrix(3,4)/2  Setx0=off  InitialVoltage=0  Measurements=None
  Ccs2/2 : powerlib/Elements/Series RLC Branch  LConnTagsString=__new0  RConnTagsString=__new0  BranchType=C  Resistance=190  Inductance=1e-3  SetiL0=off  InitialCurrent=0  Capacitance=-C_matrix(3,4)/2  Setx0=off  InitialVoltage=0  Measurements=None
  Ccs2/3 : powerlib/Elements/Series RLC Branch  LConnTagsString=__new0  RConnTagsString=__new0  BranchType=R  Resistance=-Rg_matrix(3,4)*2  Inductance=1e-3  SetiL0=off  InitialCurrent=0  Capacitance=Rg_matrix(3,4)*2  Setx0=off  InitialVoltage=0  Measurements=None
  Ccs2/4 : powerlib/Elements/Series RLC Branch  LConnTagsString=__new0  RConnTagsString=__new0  BranchType=R  Resistance=-Rg_matrix(3,4)*2  Inductance=1e-3  SetiL0=off  InitialCurrent=0  Capacitance=Rg_matrix(3,4)*2  Setx0=off  InitialVoltage=0  Measurements=None
  Ccs3/1 : powerlib/Elements/Series RLC Branch  LConnTagsString=__new0  RConnTagsString=__new0  BranchType=C  Resistance=190  Inductance=1e-3  SetiL0=off  InitialCurrent=0  Capacitance=-C_matrix(5,6)/2  Setx0=off  InitialVoltage=0  Measurements=None
  Ccs3/2 : powerlib/Elements/Series RLC Branch  LConnTagsString=__new0  RConnTagsString=__new0  BranchType=C  Resistance=190  Inductance=1e-3  SetiL0=off  InitialCurrent=0  Capacitance=-C_matrix(5,6)/2  Setx0=off  InitialVoltage=0  Measurements=None
  Ccs3/3 : powerlib/Elements/Series RLC Branch  LConnTagsString=__new0  RConnTagsString=__new0  BranchType=R  Resistance=-Rg_matrix(5,6)*2  Inductance=1e-3  SetiL0=off  InitialCurrent=0  Capacitance=-C_matrix(5,6)/2  Setx0=off  InitialVoltage=0  Measurements=None
  Ccs3/4 : powerlib/Elements/Series RLC Branch  LConnTagsString=__new0  RConnTagsString=__new0  BranchType=R  Resistance=-Rg_matrix(5,6)*2  Inductance=1e-3  SetiL0=off  InitialCurrent=0  Capacitance=-C_matrix(5,6)/2  Setx0=off  InitialVoltage=0  Measurements=None
  Csg/2 : powerlib/Elements/Series RLC Branch  LConnTagsString=__new0  RConnTagsString=__new0  BranchType=C  Resistance=190  Inductance=1e-3  SetiL0=off  InitialCurrent=0  Capacitance=( C_matrix(1,2) + C_matrix(2,2) )/2  Setx0=off  InitialVoltage=0  Measurements=None
  Csg1/1 : powerlib/Elements/Series RLC Branch  LConnTagsString=__new0  RConnTagsString=__new0  BranchType=C  Resistance=190  Inductance=1e-3  SetiL0=off  InitialCurrent=0  Capacitance=( C_matrix(1,2) + C_matrix(2,2) )/2  Setx0=off  InitialVoltage=0  Measurements=None
  Csg2/1 : powerlib/Elements/Series RLC Branch  LConnTagsString=__new0  RConnTagsString=__new0  BranchType=C  Resistance=190  Inductance=1e-3  SetiL0=off  InitialCurrent=0  Capacitance=( C_matrix(3,4) + C_matrix(4,4) )/2  Setx0=off  InitialVoltage=0  Measurements=None
  Csg2/2 : powerlib/Elements/Series RLC Branch  LConnTagsString=__new0  RConnTagsString=__new0  BranchType=C  Resistance=190  Inductance=1e-3  SetiL0=off  InitialCurrent=0  Capacitance=( C_matrix(3,4) + C_matrix(4,4) )/2  Setx0=off  InitialVoltage=0  Measurements=None
  Csg3/1 : powerlib/Elements/Series RLC Branch  LConnTagsString=__new0  RConnTagsString=__new0  BranchType=C  Resistance=190  Inductance=1e-3  SetiL0=off  InitialCurrent=0  Capacitance=( C_matrix(5,6) + C_matrix(6,6) ) /2  Setx0=off  InitialVoltage=0  Measurements=None
  Csg3/2 : powerlib/Elements/Series RLC Branch  LConnTagsString=__new0  RConnTagsString=__new0  BranchType=C  Resistance=190  Inductance=1e-3  SetiL0=off  InitialCurrent=0  Capacitance=( C_matrix(5,6) + C_matrix(6,6) ) /2  Setx0=off  InitialVoltage=0  Measurements=None
  Ground{1..4} (4 alike) : powerlib/Elements/Ground  LConnTagsString=a
  RL : powerlib/Elements/Mutual Inductance  LConnTagsString=a|b|c|L4|L5|L6  RConnTagsString=A|B|C|R4|R5|R6  TypeOfMutual=Generalized mutual inductance  NumberOfWindings=6  SelfImpedance1=[1.1 1.1e-03]  SelfImpedance2=[ 1.1 1.1e-03]  ThreeWindings=on  SelfImpedance3=[ 1.1 1.1e-03]  MutualImpedance=[1.0 1.0e-03]  InductanceMatrix=L_matrix  ResistanceMatrix=R_matrix  Measurements=None
      settings: AttributesFormatString=\n
  Rcs*2 : powerlib/Elements/Series RLC Branch  LConnTagsString=__new0  RConnTagsString=__new0  BranchType=R  Resistance=-Rg_matrix(1,2)*2  Inductance=1e-3  SetiL0=off  InitialCurrent=0  Capacitance=Rg_matrix(1,2)*2  Setx0=off  InitialVoltage=0  Measurements=None
  Rgcs1/1 : powerlib/Elements/Series RLC Branch  LConnTagsString=__new0  RConnTagsString=__new0  BranchType=R  Resistance=-Rg_matrix(1,2)*2  Inductance=1e-3  SetiL0=off  InitialCurrent=0  Capacitance=Rg_matrix(1,2)*2  Setx0=off  InitialVoltage=0  Measurements=None
  Rgsg1/1 : powerlib/Elements/Series RLC Branch  LConnTagsString=__new0  RConnTagsString=__new0  BranchType=R  Resistance=(Rg_matrix(4,4)+Rg_matrix(3,4))*2  Inductance=1e-3  SetiL0=off  InitialCurrent=0  Capacitance=Rg_matrix(1,2)*2  Setx0=off  InitialVoltage=0  Measurements=None
  Rgsg1/2 : powerlib/Elements/Series RLC Branch  LConnTagsString=__new0  RConnTagsString=__new0  BranchType=R  Resistance=(Rg_matrix(2,2)+Rg_matrix(1,2))*2  Inductance=1e-3  SetiL0=off  InitialCurrent=0  Capacitance=Rg_matrix(1,2)*2  Setx0=off  InitialVoltage=0  Measurements=None
  Rgsg1/3 : powerlib/Elements/Series RLC Branch  LConnTagsString=__new0  RConnTagsString=__new0  BranchType=R  Resistance=(Rg_matrix(4,4)+Rg_matrix(3,4))*2  Inductance=1e-3  SetiL0=off  InitialCurrent=0  Capacitance=Rg_matrix(1,2)*2  Setx0=off  InitialVoltage=0  Measurements=None
  Rgsg1/4 : powerlib/Elements/Series RLC Branch  LConnTagsString=__new0  RConnTagsString=__new0  BranchType=R  Resistance=(Rg_matrix(2,2)+Rg_matrix(1,2))*2  Inductance=1e-3  SetiL0=off  InitialCurrent=0  Capacitance=Rg_matrix(1,2)*2  Setx0=off  InitialVoltage=0  Measurements=None
  Rsg*2 : powerlib/Elements/Series RLC Branch  LConnTagsString=__new0  RConnTagsString=__new0  BranchType=R  Resistance=(Rg_matrix(6,6)+Rg_matrix(5,6))*2  Inductance=1e-3  SetiL0=off  InitialCurrent=0  Capacitance=Rg_matrix(1,2)*2  Setx0=off  InitialVoltage=0  Measurements=None
  Rsg1/1 : powerlib/Elements/Series RLC Branch  LConnTagsString=__new0  RConnTagsString=__new0  BranchType=R  Resistance=(Rg_matrix(6,6)+Rg_matrix(5,6))*2  Inductance=1e-3  SetiL0=off  InitialCurrent=0  Capacitance=Rg_matrix(1,2)*2  Setx0=off  InitialVoltage=0  Measurements=None
  A : PMIOPort  Side=Left
  B : PMIOPort  Port=2  Side=Left
  C : PMIOPort  Port=3  Side=Left
  a : PMIOPort  Port=4  Side=Right
  b : PMIOPort  Port=5  Side=Right
  c : PMIOPort  Port=6  Side=Right
  connections:
  RL/LConn6 -- Ground3/LConn1 -- Rgsg1/2/LConn1 -- Csg/2/LConn1 -- Rcs*2/LConn1 -- Ccs/2/LConn1 -- RL/LConn2 -- RL/LConn4 -- Rgsg1/1/LConn1 -- Csg2/2/LConn1 -- Ccs2/3/LConn1 -- Ccs2/2/LConn1 -- Rsg*2/LConn1 -- Csg3/2/LConn1 -- Ccs3/3/LConn1 -- Ccs3/2/LConn1
  Rsg1/1/RConn1 -- Rgsg1/3/RConn1 -- Rgsg1/4/RConn1 -- Csg3/1/RConn1 -- Csg2/1/RConn1 -- Ground2/LConn1 -- Csg1/1/RConn1
  Rgsg1/3/LConn1 -- Ccs2/4/LConn1 -- Csg2/1/LConn1 -- Ccs2/1/LConn1 -- RL/RConn4 -- Rgsg1/4/LConn1 -- Rgcs1/1/LConn1 -- Csg1/1/LConn1 -- Ccs/1/LConn1 -- RL/RConn2 -- Ground4/LConn1 -- RL/RConn6 -- Ccs3/1/LConn1 -- Rsg1/1/LConn1 -- Ccs3/4/LConn1 -- Csg3/1/LConn1
  Rsg*2/RConn1 -- Rgsg1/1/RConn1 -- Rgsg1/2/RConn1 -- Csg3/2/RConn1 -- Csg2/2/RConn1 -- Ground1/LConn1 -- Csg/2/RConn1
  a/RConn1 -- RL/RConn1 -- Rgcs1/1/RConn1 -- Ccs/1/RConn1
  b/RConn1 -- RL/RConn3 -- Ccs2/4/RConn1 -- Ccs2/1/RConn1
  Ccs3/1/RConn1 -- c/RConn1 -- RL/RConn5 -- Ccs3/4/RConn1
  RL/LConn1 -- A/RConn1 -- Rcs*2/RConn1 -- Ccs/2/RConn1
  RL/LConn3 -- B/RConn1 -- Ccs2/3/RConn1 -- Ccs2/2/RConn1
  Ccs3/2/RConn1 -- C/RConn1 -- RL/LConn5 -- Ccs3/3/RConn1
